simulink model "calcola_A2"  (R2017a)
settings: Solver=FixedStepAuto  StartTime=0.0  StopTime=80  FixedStep=Tc  RelTol=1e-3
libraries: cstblocks x1
settings Model: Creator=Enrico Donato  LastModifiedBy=Enrico Donato

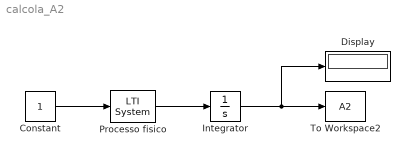
== system calcola_A2 ==
  Constant : Constant
  Display : Display
  Integrator : Integrator
  Processo fisico : cstblocks/LTI System  sys=G  IC=[]
  To Workspace2 : ToWorkspace  VariableName=A2  SampleTime=-1
  wires:
  Constant/1 -> Processo fisico/1
  Processo fisico/1 -> Integrator/1
  Integrator/1 -> Display/1, To Workspace2/1
